simulink model "Control_Potencia_cascada"  (R2023b)
settings: Solver=FixedStepAuto  StartTime=0.0  StopTime=20  FixedStep=0.01  RelTol=1e-9  EnableMultiTasking=on
libraries: arduinolib x24, slpidlib x4, dspfdesign x1, simulink x1
settings Model: SimulationMode=external  ExtModeTrigDuration=2  Creator=Juan F  LastModifiedBy=ACER
settings DataIOCC: ReturnWorkspaceOutputs=off
settings OptimizationCC: EnhancedBackFolding=on  PassReuseOutputArgsAs=Individual arguments  ZeroExternalMemoryAtStartup=off  ZeroInternalMemoryAtStartup=off  MaxStackSize=64  OptimizeBlockOrder=speed  DifferentSizesBufferReuse=on  EfficientTunableParamExpr=on
settings DebuggingCC: AlgebraicLoopMsg=none  ParameterTunabilityLossMsg=error  UnconnectedInputMsg=warning  UnconnectedOutputMsg=warning  UnconnectedLineMsg=warning
settings HardwareCC: ProdBitPerInt=16  ProdBitPerPointer=16  ProdBitPerSizeT=16  ProdBitPerPtrDiffT=16  ProdLargestAtomicFloat=None  ProdWordSize=8  ProdHWDeviceType=Atmel->AVR
settings ModelReferenceCC: EnableRefExpFcnMdlSchedulingChecks=on  ModelReferenceMinAlgLoopOccurrences=on
settings SFSimCC: MATLABDynamicMemAlloc=off  CustomCodeUndefinedFunction=UseInterfaceOnly
settings RTWCC: Description=Embedded Coder  SystemTargetFile=ert.tlc  HardwareBoard=Arduino Mega 2560  TemplateMakefile=ert_default_tmf  Toolchain=Arduino AVR  BuildConfiguration=Faster Runs
settings CodeAppCC: ForceParamTrailComments=on  IgnoreCustomStorageClasses=off  OperatorAnnotations=on  SimulinkDataObjDesc=on  SFDataObjDesc=on  InsertBlockDesc=on
settings ERTTargetCC: SupportContinuousTime=on  SupportNonInlinedSFcns=on  SupportVariableSizeSignals=on  ExtMode=on  ExtModeTransport=3  ExtModeStaticAlloc=on  ExtModeStaticAllocSize=2048  ExtModeMexFile=ext_xcp  ExtModeMexArgs=0 5 921600  ExtModeIntrfLevel=Level2 - Open

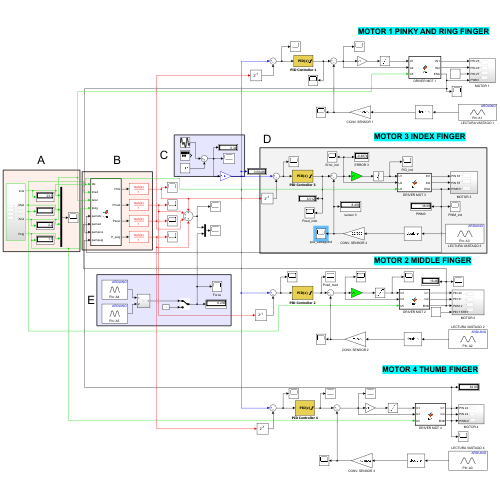
[thumbnail: Simulink's stored preview of the top-level diagram]
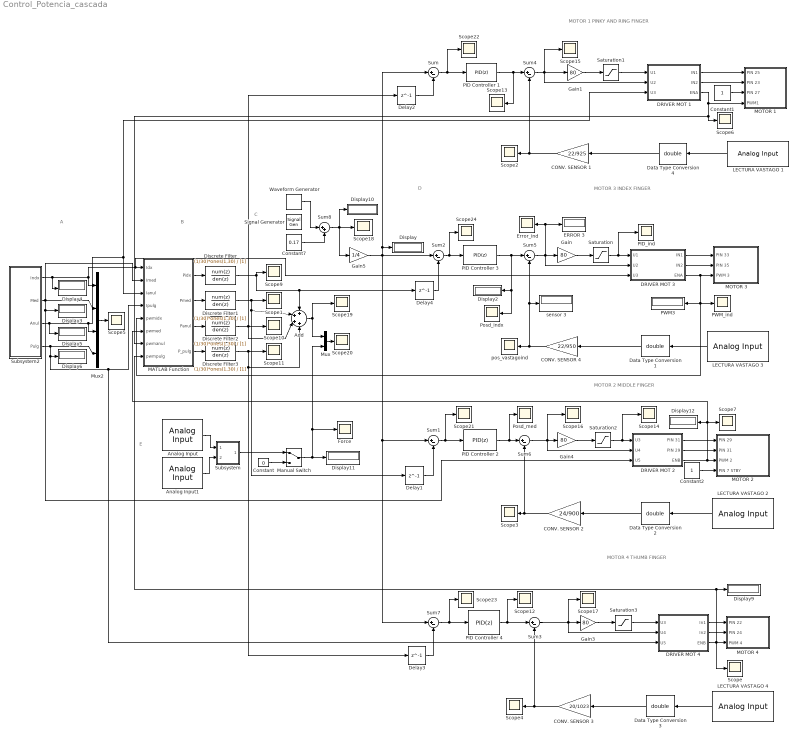
== system Control_Potencia_cascada ==
  note: A
  note: MOTOR 2 MIDDLE FINGER
  note: MOTOR 1 PINKY AND RING FINGER
  note: MOTOR 3 INDEX FINGER
  note: MOTOR 4 THUMB FINGER
  note: B
  note: C
  note: D
  note: E
  Add : Sum  Inputs=++++
  Analog Input : arduinolib/Analog Input  pinNumber=4  ReadResultsOnly=off  ConversionTriggerSource=Software  ExternalTriggerType=uint32(0)  OutputDataType=uint16  EnableConversionCompleteNotify=off  EnableOuputStatus=off  SampleTime=0.01  blockPlatform=arduino
  Analog Input1 : arduinolib/Analog Input  pinNumber=5  ReadResultsOnly=off  ConversionTriggerSource=Software  ExternalTriggerType=uint32(0)  OutputDataType=uint16  EnableConversionCompleteNotify=off  EnableOuputStatus=off  SampleTime=0.01  blockPlatform=arduino
  CONV. SENSOR 1 : Gain  Gain=22/925  OutDataTypeStr=double
  CONV. SENSOR 2 : Gain  Gain=24/900  OutDataTypeStr=double
  CONV. SENSOR 3 : Gain  Gain=20/1023  OutDataTypeStr=double
  CONV. SENSOR 4 : Gain  Gain=22/950  OutDataTypeStr=double
  Constant : Constant  Value=0
  Constant1 : Constant
  Constant2 : Constant
  Constant7 : Constant  Value=0.17  SampleTime=0.01
  DRIVER MOT 1 : MATLAB Function  TreatAsAtomicUnit=on
  DRIVER MOT 2 : MATLAB Function  TreatAsAtomicUnit=on
  DRIVER MOT 3 : MATLAB Function  TreatAsAtomicUnit=on
  DRIVER MOT 4 : MATLAB Function  TreatAsAtomicUnit=on
  Data Type Conversion{1..4} (4 alike) : DataTypeConversion  OutDataTypeStr=double  SaturateOnIntegerOverflow=off  RndMeth=Floor
  Delay{1..4} (4 alike) : Delay  DelayLength=1  SampleTime=0.01
  Discrete Filter{,1..3} (4 alike) : DiscreteFilter  Numerator=(1/30)*ones(1,30)  Denominator=[1]
  Display{,2..6,9..12} (10 alike) : Display
  ERROR 3 : Display
  Error_ind : Scope
  Force : Scope
  Gain{,1,3..4} (4 alike) : Gain  Gain=80
  Gain5 : Gain  Gain=1/4
  LECTURA VASTAGO 1 : arduinolib/Analog Input  pinNumber=1  ReadResultsOnly=off  ConversionTriggerSource=Software  ExternalTriggerType=uint32(0)  OutputDataType=uint16  EnableConversionCompleteNotify=off  EnableOuputStatus=off  SampleTime=0.01  blockPlatform=arduino
  LECTURA VASTAGO 2 : arduinolib/Analog Input  pinNumber=2  ReadResultsOnly=off  ConversionTriggerSource=Software  ExternalTriggerType=uint32(0)  OutputDataType=uint16  EnableConversionCompleteNotify=off  EnableOuputStatus=off  SampleTime=0.01  blockPlatform=arduino
  LECTURA VASTAGO 3 : arduinolib/Analog Input  pinNumber=3  ReadResultsOnly=off  ConversionTriggerSource=Software  ExternalTriggerType=uint32(0)  OutputDataType=uint16  EnableConversionCompleteNotify=off  EnableOuputStatus=off  SampleTime=0.01  blockPlatform=arduino
  LECTURA VASTAGO 4 : arduinolib/Analog Input  pinNumber=0  ReadResultsOnly=off  ConversionTriggerSource=Software  ExternalTriggerType=uint32(0)  OutputDataType=uint16  EnableConversionCompleteNotify=off  EnableOuputStatus=off  SampleTime=0.01  blockPlatform=arduino
  MATLAB Function : MATLAB Function  TreatAsAtomicUnit=on
  "MOTOR 1 " : Subsystem
  MOTOR 2 : Subsystem
  MOTOR 3 : Subsystem
  MOTOR 4 : Subsystem
  Manual Switch : ManualSwitch
  Mux : Mux  Inputs=2
  Mux2 : Mux
  PID Controller 1 : slpidlib/PID Controller  Controller=PID  Form=Parallel  TimeDomain=Discrete-time  UseExternalTs=off  SampleTime=0.01  IntegratorMethod=Trapezoidal  FilterMethod=Trapezoidal  ControllerParametersSource=internal  P=-55  I=0.01  UseKiTs=off  D=0.1  N=10  UseFilter=on  TunerSelectOption=Transfer Function Based (PID Tuner App)  InitialConditionSource=internal  InitialConditionForIntegrator=8  InitialConditionForFilter=8  DifferentiatorICPrevScaledInput=0  ExternalReset=none  TrackingMode=off  Kt=1  LimitOutput=on  SatLimitsSource=internal  UpperSaturationLimit=9.5  LowerSaturationLimit=7.5  LinearizeAsGain=off  AntiWindupMode=back-calculation  Kb=1  LimitIntegrator=off  UpperIntegratorSaturationLimit=inf  LowerIntegratorSaturationLimit=-inf  POutMin=[]  POutMax=[]  IOutMin=[]  IOutMax=[]  DOutMin=[]  DOutMax=[]  NOutMin=[]  NOutMax=[]  SumOutMin=[]  SumOutMax=[]  SaturationOutMin=[]  SaturationOutMax=[]  PParamMin=[]  PParamMax=[]  IParamMin=[]  IParamMax=[]  DParamMin=[]  DParamMax=[]  NParamMin=[]  NParamMax=[]  KbParamMin=[]  KbParamMax=[]  KtParamMin=[]  KtParamMax=[]  KbOutMin=[]  KbOutMax=[]  KtOutMin=[]  KtOutMax=[]  IntegratorOutMin=[]  IntegratorOutMax=[]  FilterOutMin=[]  FilterOutMax=[]  SumI1OutMin=[]  SumI1OutMax=[]  SumI2OutMin=[]  SumI2OutMax=[]  SumI3OutMin=[]  SumI3OutMax=[]  SumI4OutMin=[]  SumI4OutMax=[]  SumDOutMin=[]  SumDOutMax=[]  DifferentiatorOutMin=[]  DifferentiatorOutMax=[]  FilterDiffOutCoefMin=[]  FilterDiffOutCoefMax=[]  ReciprocalOutMin=[]  ReciprocalOutMax=[]  SumDenOutMin=[]  SumDenOutMax=[]  SumNumOutMin=[]  SumNumOutMax=[]  DivideOutMin=[]  DivideOutMax=[]  UdiffTsProdOutMin=[]  UdiffTsProdOutMax=[]  NTsProdOutMin=[]  NTsProdOutMax=[]  UintegralTsProdOutMin=[]  UintegralTsProdOutMax=[]  UngainTsProdOutMin=[]  UngainTsProdOutMax=[]  ClampingZeroOutDataTypeStr=Inherit: Inherit via back propagation  ClampingZeroOutMin=[]  ClampingZeroOutMax=[]  FilterDenConstantOutDataTypeStr=Inherit: Inherit via back propagation  FilterDenConstantOutMin=[]  FilterDenConstantOutMax=[]  PCopyOutDataTypeStr=Inherit: Inherit via back propagation  PCopyOutMin=[]  PCopyOutMax=[]  NCopyOutDataTypeStr=Inherit: Inherit via back propagation  NCopyOutMin=[]  NCopyOutMax=[]  IntegratorContinuousStateAttributes=''  IntegratorStateMustResolveToSignalObject=off  IntegratorRTWStateStorageClass=Auto  FilterContinuousStateAttributes=''  FilterStateMustResolveToSignalObject=off  FilterRTWStateStorageClass=Auto  ParallelPVariant=InternalParameters  IdealPVariant=Disabled  IVariant=InternalParameters  DVariant=InternalParameters  IntegratorVariant=Discrete  SatVariant=Enabled  AWVariant=BackCalculation  PCopyVariant=Disabled  TRVariant=Disabled  FdbkBlocksVariant=Feedback  IdealPFdbkVariant=Passthrough  SatFdbkVariant=Enabled  DerivativeFilterVariant=TrapezoidalFilter  NVariant=InternalParameters  NCopyVariant=InternalParameters  FilterICVariant=InternalICsFilter  IntegratorICVariant=InternalICs  ExternalResetVariant=Disabled  TRSumVariant=Passthrough  SumFdbkVariant=Enabled  SumVariant=Sum_PID  TsampFilterVariant=InternalTs  TsampNgainVariant=Passthrough  TsampIntegralVariant=Disabled_SignalSpec  ExternalSaturationOutDataTypeStr=Inherit: Same as second input
  PID Controller 2 : slpidlib/PID Controller  Controller=PID  Form=Parallel  TimeDomain=Discrete-time  UseExternalTs=off  SampleTime=0.01  IntegratorMethod=Trapezoidal  FilterMethod=Trapezoidal  ControllerParametersSource=internal  P=-40  I=0.01  UseKiTs=off  D=0.1  N=10  UseFilter=on  TunerSelectOption=Transfer Function Based (PID Tuner App)  InitialConditionSource=internal  InitialConditionForIntegrator=8  InitialConditionForFilter=8  DifferentiatorICPrevScaledInput=0  ExternalReset=none  TrackingMode=off  Kt=1  LimitOutput=on  SatLimitsSource=internal  UpperSaturationLimit=9.5  LowerSaturationLimit=7.5  LinearizeAsGain=off  AntiWindupMode=back-calculation  Kb=1  LimitIntegrator=off  UpperIntegratorSaturationLimit=inf  LowerIntegratorSaturationLimit=-inf  POutMin=[]  POutMax=[]  IOutMin=[]  IOutMax=[]  DOutMin=[]  DOutMax=[]  NOutMin=[]  NOutMax=[]  SumOutMin=[]  SumOutMax=[]  SaturationOutMin=[]  SaturationOutMax=[]  PParamMin=[]  PParamMax=[]  IParamMin=[]  IParamMax=[]  DParamMin=[]  DParamMax=[]  NParamMin=[]  NParamMax=[]  KbParamMin=[]  KbParamMax=[]  KtParamMin=[]  KtParamMax=[]  KbOutMin=[]  KbOutMax=[]  KtOutMin=[]  KtOutMax=[]  IntegratorOutMin=[]  IntegratorOutMax=[]  FilterOutMin=[]  FilterOutMax=[]  SumI1OutMin=[]  SumI1OutMax=[]  SumI2OutMin=[]  SumI2OutMax=[]  SumI3OutMin=[]  SumI3OutMax=[]  SumI4OutMin=[]  SumI4OutMax=[]  SumDOutMin=[]  SumDOutMax=[]  DifferentiatorOutMin=[]  DifferentiatorOutMax=[]  FilterDiffOutCoefMin=[]  FilterDiffOutCoefMax=[]  ReciprocalOutMin=[]  ReciprocalOutMax=[]  SumDenOutMin=[]  SumDenOutMax=[]  SumNumOutMin=[]  SumNumOutMax=[]  DivideOutMin=[]  DivideOutMax=[]  UdiffTsProdOutMin=[]  UdiffTsProdOutMax=[]  NTsProdOutMin=[]  NTsProdOutMax=[]  UintegralTsProdOutMin=[]  UintegralTsProdOutMax=[]  UngainTsProdOutMin=[]  UngainTsProdOutMax=[]  ClampingZeroOutDataTypeStr=Inherit: Inherit via back propagation  ClampingZeroOutMin=[]  ClampingZeroOutMax=[]  FilterDenConstantOutDataTypeStr=Inherit: Inherit via back propagation  FilterDenConstantOutMin=[]  FilterDenConstantOutMax=[]  PCopyOutDataTypeStr=Inherit: Inherit via back propagation  PCopyOutMin=[]  PCopyOutMax=[]  NCopyOutDataTypeStr=Inherit: Inherit via back propagation  NCopyOutMin=[]  NCopyOutMax=[]  IntegratorContinuousStateAttributes=''  IntegratorStateMustResolveToSignalObject=off  IntegratorRTWStateStorageClass=Auto  FilterContinuousStateAttributes=''  FilterStateMustResolveToSignalObject=off  FilterRTWStateStorageClass=Auto  ParallelPVariant=InternalParameters  IdealPVariant=Disabled  IVariant=InternalParameters  DVariant=InternalParameters  IntegratorVariant=Discrete  SatVariant=Enabled  AWVariant=BackCalculation  PCopyVariant=Disabled  TRVariant=Disabled  FdbkBlocksVariant=Feedback  IdealPFdbkVariant=Passthrough  SatFdbkVariant=Enabled  DerivativeFilterVariant=TrapezoidalFilter  NVariant=InternalParameters  NCopyVariant=InternalParameters  FilterICVariant=InternalICsFilter  IntegratorICVariant=InternalICs  ExternalResetVariant=Disabled  TRSumVariant=Passthrough  SumFdbkVariant=Enabled  SumVariant=Sum_PID  TsampFilterVariant=InternalTs  TsampNgainVariant=Passthrough  TsampIntegralVariant=Disabled_SignalSpec  ExternalSaturationOutDataTypeStr=Inherit: Same as second input
  PID Controller 3 : slpidlib/PID Controller  Controller=PID  Form=Parallel  TimeDomain=Discrete-time  UseExternalTs=off  SampleTime=0.01  IntegratorMethod=Trapezoidal  FilterMethod=Trapezoidal  ControllerParametersSource=internal  P=-40  I=0.01  UseKiTs=off  D=0.1  N=10  UseFilter=on  TunerSelectOption=Frequency Response Based  InitialConditionSource=internal  InitialConditionForIntegrator=8  InitialConditionForFilter=8  DifferentiatorICPrevScaledInput=0  ExternalReset=none  TrackingMode=off  Kt=1  LimitOutput=on  SatLimitsSource=internal  UpperSaturationLimit=9.5  LowerSaturationLimit=7.5  LinearizeAsGain=off  AntiWindupMode=back-calculation  Kb=1  LimitIntegrator=off  UpperIntegratorSaturationLimit=inf  LowerIntegratorSaturationLimit=-inf  POutMin=[]  POutMax=[]  IOutMin=[]  IOutMax=[]  DOutMin=[]  DOutMax=[]  NOutMin=[]  NOutMax=[]  SumOutMin=[]  SumOutMax=[]  SaturationOutMin=[]  SaturationOutMax=[]  PParamMin=[]  PParamMax=[]  IParamMin=[]  IParamMax=[]  DParamMin=[]  DParamMax=[]  NParamMin=[]  NParamMax=[]  KbParamMin=[]  KbParamMax=[]  KtParamMin=[]  KtParamMax=[]  KbOutMin=[]  KbOutMax=[]  KtOutMin=[]  KtOutMax=[]  IntegratorOutMin=[]  IntegratorOutMax=[]  FilterOutMin=[]  FilterOutMax=[]  SumI1OutMin=[]  SumI1OutMax=[]  SumI2OutMin=[]  SumI2OutMax=[]  SumI3OutMin=[]  SumI3OutMax=[]  SumI4OutMin=[]  SumI4OutMax=[]  SumDOutMin=[]  SumDOutMax=[]  DifferentiatorOutMin=[]  DifferentiatorOutMax=[]  FilterDiffOutCoefMin=[]  FilterDiffOutCoefMax=[]  ReciprocalOutMin=[]  ReciprocalOutMax=[]  SumDenOutMin=[]  SumDenOutMax=[]  SumNumOutMin=[]  SumNumOutMax=[]  DivideOutMin=[]  DivideOutMax=[]  UdiffTsProdOutMin=[]  UdiffTsProdOutMax=[]  NTsProdOutMin=[]  NTsProdOutMax=[]  UintegralTsProdOutMin=[]  UintegralTsProdOutMax=[]  UngainTsProdOutMin=[]  UngainTsProdOutMax=[]  ClampingZeroOutDataTypeStr=Inherit: Inherit via back propagation  ClampingZeroOutMin=[]  ClampingZeroOutMax=[]  FilterDenConstantOutDataTypeStr=Inherit: Inherit via back propagation  FilterDenConstantOutMin=[]  FilterDenConstantOutMax=[]  PCopyOutDataTypeStr=Inherit: Inherit via back propagation  PCopyOutMin=[]  PCopyOutMax=[]  NCopyOutDataTypeStr=Inherit: Inherit via back propagation  NCopyOutMin=[]  NCopyOutMax=[]  IntegratorContinuousStateAttributes=''  IntegratorStateMustResolveToSignalObject=off  IntegratorRTWStateStorageClass=Auto  FilterContinuousStateAttributes=''  FilterStateMustResolveToSignalObject=off  FilterRTWStateStorageClass=Auto  ParallelPVariant=InternalParameters  IdealPVariant=Disabled  IVariant=InternalParameters  DVariant=InternalParameters  IntegratorVariant=Discrete  SatVariant=Enabled  AWVariant=BackCalculation  PCopyVariant=Disabled  TRVariant=Disabled  FdbkBlocksVariant=Feedback  IdealPFdbkVariant=Passthrough  SatFdbkVariant=Enabled  DerivativeFilterVariant=TrapezoidalFilter  NVariant=InternalParameters  NCopyVariant=InternalParameters  FilterICVariant=InternalICsFilter  IntegratorICVariant=InternalICs  ExternalResetVariant=Disabled  TRSumVariant=Passthrough  SumFdbkVariant=Enabled  SumVariant=Sum_PID  TsampFilterVariant=InternalTs  TsampNgainVariant=Passthrough  TsampIntegralVariant=Disabled_SignalSpec  ExternalSaturationOutDataTypeStr=Inherit: Same as second input
  PID Controller 4 : slpidlib/PID Controller  Controller=PID  Form=Parallel  TimeDomain=Discrete-time  UseExternalTs=off  SampleTime=0.01  IntegratorMethod=Trapezoidal  FilterMethod=Trapezoidal  ControllerParametersSource=internal  P=-40  I=0.01  UseKiTs=off  D=0.1  N=10  UseFilter=on  TunerSelectOption=Transfer Function Based (PID Tuner App)  InitialConditionSource=internal  InitialConditionForIntegrator=8  InitialConditionForFilter=8  DifferentiatorICPrevScaledInput=0  ExternalReset=none  TrackingMode=off  Kt=1  LimitOutput=on  SatLimitsSource=internal  UpperSaturationLimit=9.5  LowerSaturationLimit=7.5  LinearizeAsGain=off  AntiWindupMode=back-calculation  Kb=1  LimitIntegrator=off  UpperIntegratorSaturationLimit=inf  LowerIntegratorSaturationLimit=-inf  POutMin=[]  POutMax=[]  IOutMin=[]  IOutMax=[]  DOutMin=[]  DOutMax=[]  NOutMin=[]  NOutMax=[]  SumOutMin=[]  SumOutMax=[]  SaturationOutMin=[]  SaturationOutMax=[]  PParamMin=[]  PParamMax=[]  IParamMin=[]  IParamMax=[]  DParamMin=[]  DParamMax=[]  NParamMin=[]  NParamMax=[]  KbParamMin=[]  KbParamMax=[]  KtParamMin=[]  KtParamMax=[]  KbOutMin=[]  KbOutMax=[]  KtOutMin=[]  KtOutMax=[]  IntegratorOutMin=[]  IntegratorOutMax=[]  FilterOutMin=[]  FilterOutMax=[]  SumI1OutMin=[]  SumI1OutMax=[]  SumI2OutMin=[]  SumI2OutMax=[]  SumI3OutMin=[]  SumI3OutMax=[]  SumI4OutMin=[]  SumI4OutMax=[]  SumDOutMin=[]  SumDOutMax=[]  DifferentiatorOutMin=[]  DifferentiatorOutMax=[]  FilterDiffOutCoefMin=[]  FilterDiffOutCoefMax=[]  ReciprocalOutMin=[]  ReciprocalOutMax=[]  SumDenOutMin=[]  SumDenOutMax=[]  SumNumOutMin=[]  SumNumOutMax=[]  DivideOutMin=[]  DivideOutMax=[]  UdiffTsProdOutMin=[]  UdiffTsProdOutMax=[]  NTsProdOutMin=[]  NTsProdOutMax=[]  UintegralTsProdOutMin=[]  UintegralTsProdOutMax=[]  UngainTsProdOutMin=[]  UngainTsProdOutMax=[]  ClampingZeroOutDataTypeStr=Inherit: Inherit via back propagation  ClampingZeroOutMin=[]  ClampingZeroOutMax=[]  FilterDenConstantOutDataTypeStr=Inherit: Inherit via back propagation  FilterDenConstantOutMin=[]  FilterDenConstantOutMax=[]  PCopyOutDataTypeStr=Inherit: Inherit via back propagation  PCopyOutMin=[]  PCopyOutMax=[]  NCopyOutDataTypeStr=Inherit: Inherit via back propagation  NCopyOutMin=[]  NCopyOutMax=[]  IntegratorContinuousStateAttributes=''  IntegratorStateMustResolveToSignalObject=off  IntegratorRTWStateStorageClass=Auto  FilterContinuousStateAttributes=''  FilterStateMustResolveToSignalObject=off  FilterRTWStateStorageClass=Auto  ParallelPVariant=InternalParameters  IdealPVariant=Disabled  IVariant=InternalParameters  DVariant=InternalParameters  IntegratorVariant=Discrete  SatVariant=Enabled  AWVariant=BackCalculation  PCopyVariant=Disabled  TRVariant=Disabled  FdbkBlocksVariant=Feedback  IdealPFdbkVariant=Passthrough  SatFdbkVariant=Enabled  DerivativeFilterVariant=TrapezoidalFilter  NVariant=InternalParameters  NCopyVariant=InternalParameters  FilterICVariant=InternalICsFilter  IntegratorICVariant=InternalICs  ExternalResetVariant=Disabled  TRSumVariant=Passthrough  SumFdbkVariant=Enabled  SumVariant=Sum_PID  TsampFilterVariant=InternalTs  TsampNgainVariant=Passthrough  TsampIntegralVariant=Disabled_SignalSpec  ExternalSaturationOutDataTypeStr=Inherit: Same as second input
  PID_ind : Scope
  PWM3 : Display
  PWM_ind : Scope
  Posd_indx : Scope
  Posd_med : Scope
  Saturation{,1..3} (4 alike) : Saturate  UpperLimit=255  LowerLimit=-255
  Scope{,1..7,9..24} (24 alike) : Scope
  Signal Generator : SignalGenerator  WaveForm=square  Amplitude=0.06  Frequency=2*pi/8  Units=rad/sec
  Subsystem : Subsystem
  Subsystem2 : Subsystem
  Sum{,1..7} (8 alike) : Sum  Inputs=|+-
  Sum8 : Sum  Inputs=|++
  Waveform Generator : simulink/Sources/Waveform Generator  OutMin=[]  OutMax=[]  OutDataTypeStr=double  SelectedSignal=1  Signals=sin(0.17,2*pi/10,pi/2)  BlockNames=MultiportSwitch_6a78c393ae4c459  SampleTime=0.01
  pos_vastagoind : Scope
  sensor 3 : Display
  wires:
  CONV. SENSOR 2/1 -> Scope3/1, Sum6/2
  Sum6/1 -> DRIVER MOT 2/2(U4), Gain4/1, Scope16/1
  DRIVER MOT 4/3(ENB) -> MOTOR 4/3(PWM 4), Scope/1, Display9/1, MATLAB Function/8(pwmpulg)
  DRIVER MOT 4/2(In2) -> MOTOR 4/2(PIN 24)
  Sum4/1 -> Gain1/1, Scope15/1, DRIVER MOT 1/2(U2)
  Sum/1 -> Scope22/1, PID Controller 1/1
  Sum7/1 -> Scope23/1, PID Controller 4/1
  Saturation1/1 -> DRIVER MOT 1/1(U1)
  DRIVER MOT 4/1(In1) -> MOTOR 4/1(PIN 22)
  CONV. SENSOR 3/1 -> Scope4/1, Sum3/2
  Sum3/1 -> Gain3/1, DRIVER MOT 4/2(U4), Scope17/1
  CONV. SENSOR 1/1 -> Sum4/2, Scope2/1
  LECTURA VASTAGO 4/1 -> Data Type Conversion3/1
  DRIVER MOT 2/3(ENB) -> MATLAB Function/6(pwmed), Display12/1, Scope7/1, MOTOR 2/3(PWM 2)
  Saturation3/1 -> DRIVER MOT 4/1(U3)
  Sum1/1 -> Scope21/1, PID Controller 2/1
  LECTURA VASTAGO 2/1 -> Data Type Conversion2/1
  Saturation2/1 -> DRIVER MOT 2/1(U3), Scope14/1
  Constant1/1 -> "MOTOR 1 "/3(PIN 27)
  CONV. SENSOR 4/1 -> pos_vastagoind/1, Sum5/2, sensor 3/1
  LECTURA VASTAGO 3/1 -> Data Type Conversion1/1
  Constant2/1 -> MOTOR 2/4(PIN 7 STBY)
  DRIVER MOT 3/1(IN1) -> MOTOR 3/1(PIN 33)
  DRIVER MOT 3/2(IN2) -> MOTOR 3/2(PIN 35)
  DRIVER MOT 2/1(PIN 31) -> MOTOR 2/1(PIN 29)
  DRIVER MOT 2/2(PIN 29) -> MOTOR 2/2(PIN 31)
  Mux2/1 -> Scope5/1
  Manual Switch/1 -> Force/1, Mux/2, Display11/1
  Constant/1 -> Manual Switch/2
  Gain/1 -> Saturation/1
  Sum5/1 -> Gain/1, DRIVER MOT 3/2(U2), Error_ind/1, ERROR 3/1
  DRIVER MOT 1/3(ENA) -> "MOTOR 1 "/4(PWM1), Scope6/1, MATLAB Function/7(pwmanul)
  Subsystem2/1(Indx) -> DRIVER MOT 3/3(U3), MATLAB Function/1(Idx), Mux2/1, Display4/1
  Subsystem2/3(Anul) -> DRIVER MOT 1/3(U3), MATLAB Function/3(Ianul), Mux2/3, Display5/1
  Subsystem2/4(Pulg) -> Mux2/4, MATLAB Function/4(Ipulg), DRIVER MOT 4/3(U5), Display6/1
  Subsystem2/2(Med) -> Mux2/2, MATLAB Function/2(Imed), Display3/1, DRIVER MOT 2/3(U5)
  DRIVER MOT 3/3(ENA) -> MOTOR 3/3(PWM 3), PWM_ind/1, MATLAB Function/5(pwmidx), PWM3/1
  Discrete Filter/1 -> Add/1, Delay4/1, Scope9/1
  Discrete Filter2/1 -> Add/3, Scope10/1, Delay2/1
  Discrete Filter1/1 -> Delay1/1, Add/2, Scope1/1
  Discrete Filter3/1 -> Add/4, Delay3/1, Scope11/1
  Analog Input/1 -> Subsystem/1(In1)
  Analog Input1/1 -> Subsystem/2(In2)
  Subsystem/1(Out1) -> Manual Switch/1
  MATLAB Function/1(Pidx) -> Discrete Filter/1
  MATLAB Function/2(Pmed) -> Discrete Filter1/1
  MATLAB Function/3(Panul) -> Discrete Filter2/1
  MATLAB Function/4(P_pulg) -> Discrete Filter3/1
  LECTURA VASTAGO 1/1 -> Data Type Conversion4/1
  Data Type Conversion1/1 -> CONV. SENSOR 4/1
  Data Type Conversion2/1 -> CONV. SENSOR 2/1
  Data Type Conversion3/1 -> CONV. SENSOR 3/1
  Delay1/1 -> Sum1/2
  Add/1 -> Mux/1, Scope19/1
  DRIVER MOT 1/1(IN1) -> "MOTOR 1 "/1(PIN 25)
  DRIVER MOT 1/2(IN2) -> "MOTOR 1 "/2(PIN 23)
  Data Type Conversion4/1 -> CONV. SENSOR 1/1
  Mux/1 -> Scope20/1
  Delay2/1 -> Sum/2
  Delay3/1 -> Sum7/2
  Sum2/1 -> Scope24/1, PID Controller 3/1
  Saturation/1 -> DRIVER MOT 3/1(U1), PID_ind/1
  PID Controller 3/1 -> Posd_indx/1, Display2/1, Sum5/1
  Delay4/1 -> Sum2/2
  Gain1/1 -> Saturation1/1
  PID Controller 1/1 -> Scope13/1, Sum4/1
  Gain4/1 -> Saturation2/1
  PID Controller 2/1 -> Posd_med/1, Sum6/1
  PID Controller 4/1 -> Sum3/1, Scope12/1
  Gain3/1 -> Saturation3/1
  Constant7/1 -> Sum8/2
  Sum8/1 -> Gain5/1, Scope18/1, Display10/1
  Gain5/1 -> Display/1, Sum/1, Sum7/1, Sum1/1, Sum2/1
  Waveform Generator/1 -> Sum8/1

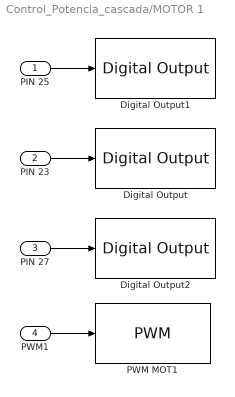
== system Control_Potencia_cascada/MOTOR 1  ==
  PIN 25 : Inport
  PIN 23 : Inport  Port=2
  PIN 27 : Inport  Port=3
  PWM1 : Inport  Port=4
  Digital Output : arduinolib/Digital Output  pinNumber=23  Direction=output  blockPlatform=arduino
  Digital Output1 : arduinolib/Digital Output  pinNumber=25  Direction=output  blockPlatform=arduino
  Digital Output2 : arduinolib/Digital Output  pinNumber=27  Direction=output  blockPlatform=arduino
  PWM MOT1 : arduinolib/PWM  pinNumber=2  frequencyType=Default  desiredFrequency=490.2  achievableFrequency=490.2
  wires:
  PWM1/1 -> PWM MOT1/1
  PIN 27/1 -> Digital Output2/1
  PIN 23/1 -> Digital Output/1
  PIN 25/1 -> Digital Output1/1

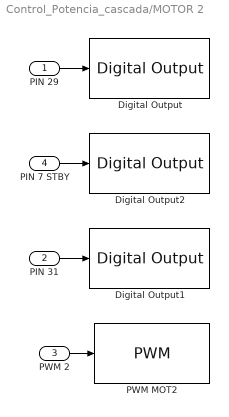
== system Control_Potencia_cascada/MOTOR 2 ==
  PIN 29 : Inport
  PIN 31 : Inport  Port=2
  PWM 2 : Inport  Port=3
  PIN 7 STBY : Inport  Port=4
  Digital Output : arduinolib/Digital Output  pinNumber=29  Direction=output  blockPlatform=arduino
  Digital Output1 : arduinolib/Digital Output  pinNumber=31  Direction=output  blockPlatform=arduino
  Digital Output2 : arduinolib/Digital Output  pinNumber=7  Direction=output  blockPlatform=arduino
  PWM MOT2 : arduinolib/PWM  pinNumber=3  frequencyType=Default  desiredFrequency=490.2  achievableFrequency=490.2
  wires:
  PWM 2/1 -> PWM MOT2/1
  PIN 29/1 -> Digital Output/1
  PIN 31/1 -> Digital Output1/1
  PIN 7 STBY/1 -> Digital Output2/1

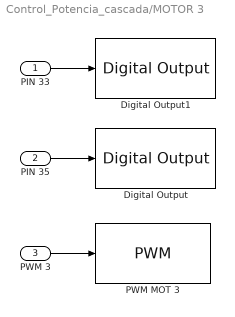
== system Control_Potencia_cascada/MOTOR 3 ==
  PIN 33 : Inport
  PIN 35 : Inport  Port=2
  PWM 3 : Inport  Port=3
  Digital Output : arduinolib/Digital Output  pinNumber=35  Direction=output  blockPlatform=arduino
  Digital Output1 : arduinolib/Digital Output  pinNumber=33  Direction=output  blockPlatform=arduino
  PWM MOT 3 : arduinolib/PWM  pinNumber=4  frequencyType=Default  desiredFrequency=490.2  achievableFrequency=490.2
  wires:
  PWM 3/1 -> PWM MOT 3/1
  PIN 35/1 -> Digital Output/1
  PIN 33/1 -> Digital Output1/1

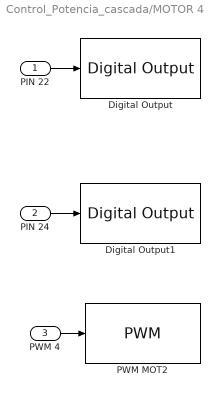
== system Control_Potencia_cascada/MOTOR 4 ==
  PIN 22 : Inport
  PIN 24 : Inport  Port=2
  PWM 4 : Inport  Port=3
  Digital Output : arduinolib/Digital Output  pinNumber=22  Direction=output  blockPlatform=arduino
  Digital Output1 : arduinolib/Digital Output  pinNumber=24  Direction=output  blockPlatform=arduino
  PWM MOT2 : arduinolib/PWM  pinNumber=5  frequencyType=Default  desiredFrequency=490.2  achievableFrequency=490.2
  wires:
  PWM 4/1 -> PWM MOT2/1
  PIN 22/1 -> Digital Output/1
  PIN 24/1 -> Digital Output1/1

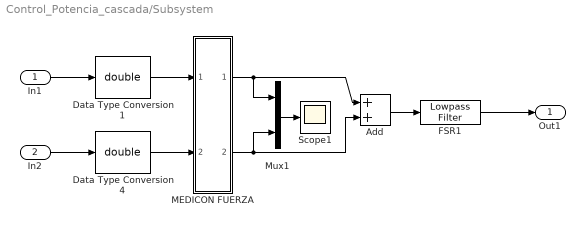
== system Control_Potencia_cascada/Subsystem ==
  In1 : Inport
  In2 : Inport  Port=2
  Add : Sum
  Data Type Conversion1 : DataTypeConversion  OutDataTypeStr=double  SaturateOnIntegerOverflow=off  RndMeth=Floor
  Data Type Conversion4 : DataTypeConversion  OutDataTypeStr=double  SaturateOnIntegerOverflow=off  RndMeth=Floor
  "FSR1 " : dspfdesign/Lowpass Filter  FilterType=FIR  DesignForMinimumOrder=on  FilterOrder=50  PassbandFrequency=5  StopbandFrequency=10  PassbandRipple=0.1  StopbandAttenuation=30  SampleRateMode=Specify on dialog  SampleRate=40  SimulateUsing=Interpreted execution  roundingMode=Floor  coeffsDataTypeStr=fixdt(1,16)
  MEDICON FUERZA : Subsystem
  Mux1 : Mux  Inputs=2
  Scope1 : Scope
  Out1 : Outport
  wires:
  MEDICON FUERZA/2(Out2) -> Add/2, Mux1/2
  Add/1 -> "FSR1 "/1
  "FSR1 "/1 -> Out1/1
  In1/1 -> Data Type Conversion1/1
  MEDICON FUERZA/1(Out1) -> Add/1, Mux1/1
  Mux1/1 -> Scope1/1
  In2/1 -> Data Type Conversion4/1
  Data Type Conversion1/1 -> MEDICON FUERZA/1(In1)
  Data Type Conversion4/1 -> MEDICON FUERZA/2(In2)

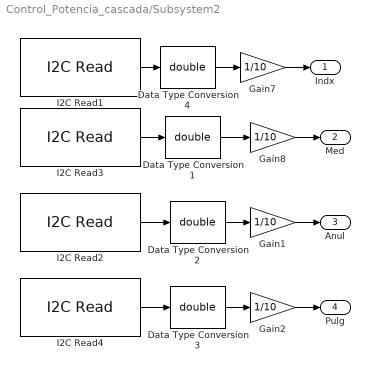
== system Control_Potencia_cascada/Subsystem2 ==
  Data Type Conversion{1..4} (4 alike) : DataTypeConversion  OutDataTypeStr=double  SaturateOnIntegerOverflow=off  RndMeth=Floor
  Gain{1..2,7..8} (4 alike) : Gain  Gain=1/10  OutDataTypeStr=double
  I2C Read1 : arduinolib/I2C Read  I2CModule=0  Mode=Master  SlaveAddress=65  SlaveByteOrder=BigEndian  Direction=Receiver  RegisterAddressMode=on  RegisterAddress=1  SlaveDataType=int16  DataLength=1  NoAck=off  RepeatedStart=off  OutputStatus=off  blockPlatform=ARDUINO  SampleTime=0.01
  I2C Read2 : arduinolib/I2C Read  I2CModule=0  Mode=Master  SlaveAddress=64  SlaveByteOrder=BigEndian  Direction=Receiver  RegisterAddressMode=on  RegisterAddress=1  SlaveDataType=int16  DataLength=1  NoAck=off  RepeatedStart=off  OutputStatus=off  blockPlatform=ARDUINO  SampleTime=0.01
  I2C Read3 : arduinolib/I2C Read  I2CModule=0  Mode=Master  SlaveAddress=68  SlaveByteOrder=BigEndian  Direction=Receiver  RegisterAddressMode=on  RegisterAddress=1  SlaveDataType=int16  DataLength=1  NoAck=off  RepeatedStart=off  OutputStatus=off  blockPlatform=ARDUINO  SampleTime=0.01
  I2C Read4 : arduinolib/I2C Read  I2CModule=0  Mode=Master  SlaveAddress=69  SlaveByteOrder=BigEndian  Direction=Receiver  RegisterAddressMode=on  RegisterAddress=1  SlaveDataType=int16  DataLength=1  NoAck=off  RepeatedStart=off  OutputStatus=off  blockPlatform=ARDUINO  SampleTime=0.01
  Indx : Outport
  Med : Outport  Port=2
  Anul : Outport  Port=3
  Pulg : Outport  Port=4
  wires:
  I2C Read1/1 -> Data Type Conversion4/1
  I2C Read3/1 -> Data Type Conversion1/1
  Gain7/1 -> Indx/1
  Gain8/1 -> Med/1
  I2C Read2/1 -> Data Type Conversion2/1
  Gain1/1 -> Anul/1
  I2C Read4/1 -> Data Type Conversion3/1
  Gain2/1 -> Pulg/1
  Data Type Conversion4/1 -> Gain7/1
  Data Type Conversion1/1 -> Gain8/1
  Data Type Conversion2/1 -> Gain1/1
  Data Type Conversion3/1 -> Gain2/1

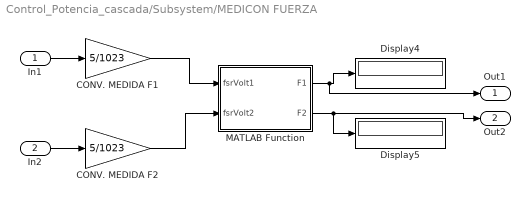
== system Control_Potencia_cascada/Subsystem/MEDICON FUERZA ==
  In1 : Inport
  In2 : Inport  Port=2
  CONV. MEDIDA F1 : Gain  Gain=5/1023  OutDataTypeStr=double  RndMeth=Round
  CONV. MEDIDA F2 : Gain  Gain=5/1023  OutDataTypeStr=double  RndMeth=Round
  Display4 : Display
      settings: Decimation=2
  Display5 : Display
      settings: Decimation=2
  MATLAB Function : MATLAB Function  TreatAsAtomicUnit=on
  Out1 : Outport  VectorParamsAs1DForOutWhenUnconnected=off
  Out2 : Outport  Port=2  VectorParamsAs1DForOutWhenUnconnected=off
  wires:
  In2/1 -> CONV. MEDIDA F2/1
  MATLAB Function/2(F2) -> Out2/1, Display5/1
  CONV. MEDIDA F2/1 -> MATLAB Function/2(fsrVolt2)
  MATLAB Function/1(F1) -> Out1/1, Display4/1
  In1/1 -> CONV. MEDIDA F1/1
  CONV. MEDIDA F1/1 -> MATLAB Function/1(fsrVolt1)

== matlab function Control_Potencia_cascada/DRIVER MOT 2 ==
  data: U3 input; In1 output; In2 output; ENB output; U4 input; U5 input
function [In1, In2, ENB] = fcn(U3,U4,U5)

if U3 > 0

    In1 = 0; % 1
    In2 = 1; % 0
    ENB = abs(U3);
    % STBY1 =1;


elseif U3 < 0

    In1 = 1;  % 0
    In2 = 0;  % 1
    ENB = abs(U3);
    %   STBY1 =1;


else
    In1 = 0;
    In2 = 0;
    ENB = 0;
end

if U4 == 0

    In1 = 0;
    In2 = 0;
    ENB = 0;
end

if abs(U5)> 180
    In1 = 0;
    In2 = 0;
    ENB = 0;

end
end

== matlab function Control_Potencia_cascada/DRIVER MOT 1 ==
  data: U1 input; IN1 output; IN2 output; ENA output; U2 input; U3 input
function [IN1, IN2, ENA] = fcn(U1,U2,U3)

     
if U1 > 0
    
    IN1 = 1; % 0
    IN2 = 0; % 1 
   
    ENA = abs(U1);
    
    
elseif U1 < 0
       
       IN1 = 0; % 1
       IN2 = 1; % 0
      
      ENA = abs(U1);
    

else
       IN1 = 0;
       IN2 = 0; 
       ENA = 0;
       
end
if U2 == 0
     
       IN1 = 0;
       IN2 = 0; 
       ENA = 0;
      
end

 if abs(U3)> 185
       IN1 = 0;
       IN2 = 0; 
       ENA = 0;
      
 end
end

== matlab function Control_Potencia_cascada/MATLAB Function ==
  data: Idx input; Pidx output; Imed input; Ianul input; Pmed output; Panul output; Ipulg input; pwmidx input; pwmed input; pwmanul input; pwmpulg input; P_pulg output
function [Pidx,Pmed,Panul,P_pulg] = fcn(Idx, Imed,Ianul,Ipulg,pwmidx,pwmed,pwmanul,pwmpulg)


Pidx = (Idx/1000)*(pwmidx*(12/255));
if Pidx < 0
    Pidx = 0;
end
Pmed = (Imed/1000)*(pwmed*(12/255));
if Pmed < 0
    Pmed = 0;
end
Panul = (Ianul/1000)*(pwmanul*(12/255));
if Panul < 0
    Panul = 0;
end

P_pulg = (Ipulg/1000)*(pwmpulg*(12/255));
if P_pulg < 0
    P_pulg = 0;
end

end

== matlab function Control_Potencia_cascada/DRIVER MOT 3 ==
  data: U1 input; IN1 output; IN2 output; ENA output; U2 input; U3 input
function [IN1, IN2, ENA] = fcn(U1,U2,U3)

if U1 > 0
    
    IN1 = 1;
    IN2 = 0;
   
    ENA = abs(U1);
    
    
elseif U1 < 0
       
       IN1 = 0;
       IN2 = 1; 
      
      ENA = abs(U1);
    

else
       IN1 = 0;
       IN2 = 0; 
       ENA = 0;
    
end
if U2 == 0
     
       IN1 = 0;
       IN2 = 0; 
       ENA = 0;
    
end

if abs(U3)> 180
       IN1 = 0;
       IN2 = 0; 
       ENA = 0;
       
 end
end

== matlab function Control_Potencia_cascada/Subsystem/MEDICON FUERZA/MATLAB Function ==
  data: fsrVolt1 input; F1 output; fsrVolt2 input; F2 output
function [F1,F2] = fcn(fsrVolt1,fsrVolt2)

% Power Curve Fit (power1)
%    f(x) = a*x^b

% FSR1
 a = 0.6275;
 b = 2.3215;

% FSR2
 a2 = 1.3997;
 b2 = 1.9536;


F1 = a * (fsrVolt1^b);
F2 = a2 * (fsrVolt2 ^b2);

== matlab function Control_Potencia_cascada/DRIVER MOT 4 ==
  data: U3 input; In1 output; In2 output; ENB output; U4 input; U5 input
function [In1, In2, ENB] = fcn(U3,U4,U5)

if U3 > 0
 
    In1 = 0; %1
    In2 = 1;
   ENB = abs(U3);
   % STBY1 =1;


elseif U3 < 0
     
       In1 = 1; %0
       In2 = 0; 
      ENB = abs(U3);
    %   STBY1 =1;
    
   
else
       In1 = 0;
       In2 = 0;  
       ENB = 0;
end

if U4 == 0
   
       In1 = 0;
       In2 = 0;  
       ENB = 0;
end

if abs(U5)> 180
       In1 = 0;
       In2 = 0; 
       ENB = 0;
       
 end
end
